simulink model "PEArray_func_sim"  (R2021a)
settings: Solver=VariableStepAuto  StartTime=0.0  StopTime=15  RelTol=1e-3
libraries: hdlBasic x164, xbsIndex_r4 x1
(part 1 of 2)
settings Model: Creator=lisix  LastModifiedBy=sl186
settings DebuggingCC: UnconnectedInputMsg=none  UnconnectedOutputMsg=none  UnconnectedLineMsg=none
settings RTWCC: DLArmComputeVersion=20.02.1

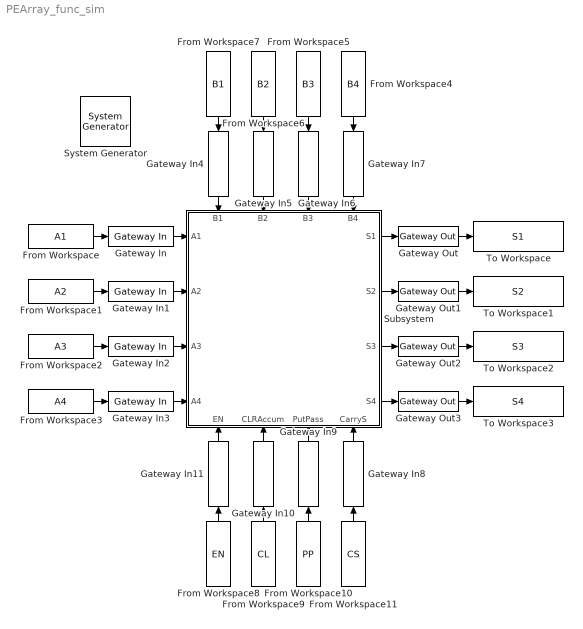
== system PEArray_func_sim ==
  " System Generator" : xbsIndex_r4/ System Generator  Tag=genX  xilinxfamily=zynq  part=xc7z020  speed=-1  package=clg484  synthesis_tool=Vivado  clock_wrapper=Clock Enables  directory=./netlist  proj_type=Vivado  Synth_file=Vivado Synthesis Defaults  Impl_file=Vivado Implementation Defaults  testbench=off  simulink_period=1  sysclk_period=10  dcm_input_clock_period=10  incr_netlist=off  trim_vbits=Everywhere in SubSystem  dbl_ovrd=According to Block Masks  core_generation=According to Block Masks  run_coregen=off  deprecated_control=off  eval_field=0  block_type=sysgen
  From Workspace : FromWorkspace  VariableName=A1  OutputAfterFinalValue=Setting to zero
  From Workspace1 : FromWorkspace  VariableName=A2  OutputAfterFinalValue=Setting to zero
  From Workspace10 : FromWorkspace  VariableName=PP  OutputAfterFinalValue=Setting to zero
  From Workspace11 : FromWorkspace  VariableName=CS  OutputAfterFinalValue=Setting to zero
  From Workspace2 : FromWorkspace  VariableName=A3  OutputAfterFinalValue=Setting to zero
  From Workspace3 : FromWorkspace  VariableName=A4  OutputAfterFinalValue=Setting to zero
  From Workspace4 : FromWorkspace  VariableName=B4  OutputAfterFinalValue=Setting to zero
  From Workspace5 : FromWorkspace  VariableName=B3  OutputAfterFinalValue=Setting to zero
  From Workspace6 : FromWorkspace  VariableName=B2  OutputAfterFinalValue=Setting to zero
  From Workspace7 : FromWorkspace  VariableName=B1  OutputAfterFinalValue=Setting to zero
  From Workspace8 : FromWorkspace  VariableName=EN  OutputAfterFinalValue=Setting to zero
  From Workspace9 : FromWorkspace  VariableName=CL  OutputAfterFinalValue=Setting to zero
  Gateway In{,1..7} (8 alike) : hdlBasic/Gateway In  gui_display_data_type=Fixed-point  arith_type=Signed (2's comp)  n_bits=16  bin_pt=10  preci_type=Single  exp_width=8  frac_width=24  rows=1  columns=1  quantization="Round  (unbiased: +/- Inf)"  overflow=Saturate  period=1  UseAsADC=off  ADCChannel='1'  interface=None  automatic_assignment=on  address_offset=hex2dec('00')  intf_name=''  intf_description=''  default_value=0  timing_constraint=None  locs_specified=off  LOCs={}  io_standard={}  inherit_from_input=off  hdl_port=on  XmcBlockStatus=1  maskContainerNames=group4  block_type=gatewayin  block_config=sysgen:gateway_in_config  block_width_w=590  block_height_w=620  block_width=640  block_height=850
  Gateway In{8..11} (4 alike) : hdlBasic/Gateway In  gui_display_data_type=Boolean  arith_type=Boolean  n_bits=16  bin_pt=10  preci_type=Single  exp_width=8  frac_width=24  rows=1  columns=1  quantization="Round  (unbiased: +/- Inf)"  overflow=Saturate  period=1  UseAsADC=off  ADCChannel='1'  interface=None  automatic_assignment=on  address_offset=hex2dec('00')  intf_name=''  intf_description=''  default_value=0  timing_constraint=None  locs_specified=off  LOCs={}  io_standard={}  inherit_from_input=off  hdl_port=on  XmcBlockStatus=1  maskContainerNames=group4  block_type=gatewayin  block_config=sysgen:gateway_in_config  block_width_w=590  block_height_w=620  block_width=640  block_height=850
  Gateway Out{,1..3} (4 alike) : hdlBasic/Gateway Out  inherit_from_input=off  hdl_port=on  rows=1  columns=1  UseAsDAC=off  DACChannel='1'  interface=None  automatic_assignment=on  address_offset=hex2dec('00')  intf_name=''  intf_description=''  timing_constraint=None  locs_specified=off  LOCs={}  io_standard={}  XmcBlockStatus=1  maskContainerNames=group4  block_type=gatewayout  block_config=sysgen:gateway_out_config  block_width_w=590  block_height_w=620  block_width=620  block_height=750
  Subsystem : Subsystem
      settings: PortSchema="{\"entries\":[{\"content\":{\"sides\":[{\"content\":{\"connectorIds\":[\"In1\",\"In2\",\"In3\",\"In4\"]},\"type\":\"ConnectorPlacement.EquallySpacedRectSide\",\"uuid\":\"ef644a02-469b-4d5d-af2f-26c489a3c425\"},{\"content\":{\"connectorIds\":[\"Out1\",\"Out2\",\"Out3\",\"Out4\"],\"side\":\"RIGHT\"},\"type\":\"ConnectorPlacement.EquallySpacedRectSide\",\"uuid\":\"314a2994-7795-41ba-894c-92e5f23e8912\"},{\"content\":{\"connectorIds\":[\"In5\",\"In6\",\"In7\",\"In8\"],\"side\":\"TOP\"},\"type\":\"ConnectorPlacement.EquallySpacedRectSide\",\"uuid\":\"0fc87e02-f682-470c-ba3d-89d91916b1fa\"},{\"content\":{\"connectorIds\":[\"In9\",\"In10\",\"In11\",\"In12\"],\"side\":\"BOTTOM\"},\"type\":\"ConnectorPlacement.EquallySpacedRectSide\",\"uuid\":\"d64b1621-eab0-4c50-9294-0c88aed07ecf\"}]},\"type\":\"ConnectorPlacement.EquallySpacedConnector\",\"uuid\":\"b7a51112-d4eb-4f46-8167-08a9d75329ad\"}],\"packageUris\":[\"http://schema.mathworks.com/mf0/Connector/R2020b\"],\"version\":\"1.0\"}"
  To Workspace : ToWorkspace  VariableName=S1  SaveFormat=Timeseries  SampleTime=-1
  To Workspace1 : ToWorkspace  VariableName=S2  SaveFormat=Timeseries  SampleTime=-1
  To Workspace2 : ToWorkspace  VariableName=S3  SaveFormat=Timeseries  SampleTime=-1
  To Workspace3 : ToWorkspace  VariableName=S4  SaveFormat=Timeseries  SampleTime=-1
  wires:
  Subsystem/1(S1) -> Gateway Out/1
  Subsystem/2(S2) -> Gateway Out1/1
  Subsystem/4(S4) -> Gateway Out3/1
  Subsystem/3(S3) -> Gateway Out2/1
  Gateway In/1 -> Subsystem/1(A1)
  Gateway In1/1 -> Subsystem/2(A2)
  Gateway In2/1 -> Subsystem/3(A3)
  Gateway In3/1 -> Subsystem/4(A4)
  Gateway In4/1 -> Subsystem/5(B1)
  Gateway In5/1 -> Subsystem/6(B2)
  Gateway In6/1 -> Subsystem/7(B3)
  Gateway In7/1 -> Subsystem/8(B4)
  From Workspace/1 -> Gateway In/1
  Gateway In11/1 -> Subsystem/9(EN)
  Gateway In10/1 -> Subsystem/10(CLRAccum)
  Gateway In9/1 -> Subsystem/11(PutPass)
  Gateway In8/1 -> Subsystem/12(CarryS)
  Gateway Out/1 -> To Workspace/1
  Gateway Out1/1 -> To Workspace1/1
  Gateway Out2/1 -> To Workspace2/1
  Gateway Out3/1 -> To Workspace3/1
  From Workspace1/1 -> Gateway In1/1
  From Workspace2/1 -> Gateway In2/1
  From Workspace3/1 -> Gateway In3/1
  From Workspace7/1 -> Gateway In4/1
  From Workspace6/1 -> Gateway In5/1
  From Workspace5/1 -> Gateway In6/1
  From Workspace4/1 -> Gateway In7/1
  From Workspace8/1 -> Gateway In11/1
  From Workspace9/1 -> Gateway In10/1
  From Workspace10/1 -> Gateway In9/1
  From Workspace11/1 -> Gateway In8/1

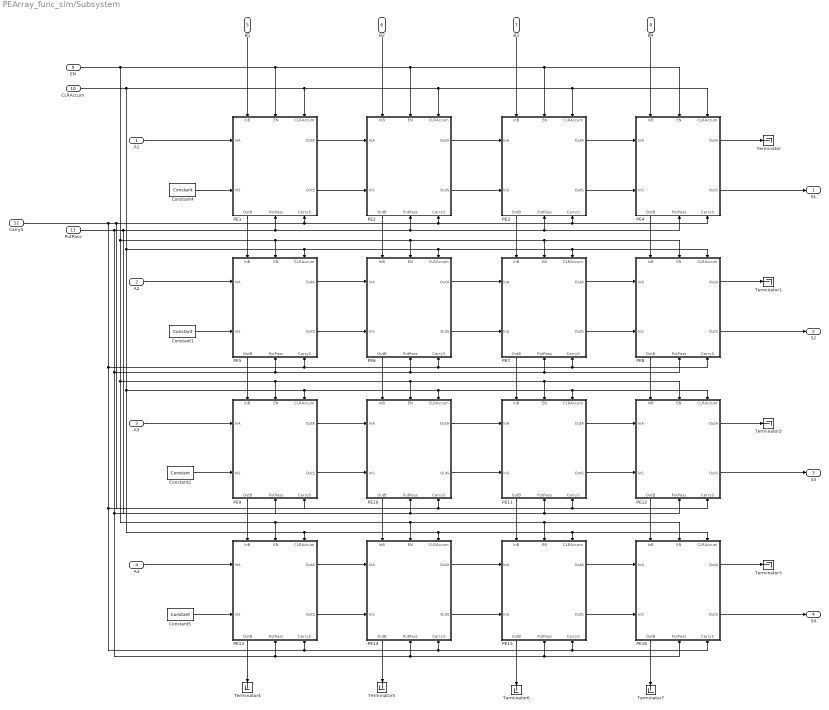
== system PEArray_func_sim/Subsystem ==
  A1 : Inport
  A2 : Inport  Port=2
  A3 : Inport  Port=3
  A4 : Inport  Port=4
  B1 : Inport  Port=5
  B2 : Inport  Port=6
  B3 : Inport  Port=7
  B4 : Inport  Port=8
  EN : Inport  Port=9
  CLRAccum : Inport  Port=10
  PutPass : Inport  Port=11
  CarryS : Inport  Port=12
  Constant{1..2,4..5} (4 alike) : hdlBasic/Constant  const=0  gui_display_data_type=Fixed-point  arith_type=Signed (2's comp)  n_bits=16  bin_pt=10  preci_type=Single  exp_width=8  frac_width=24  explicit_period=off  period=1  XmcBlockStatus=1  maskContainerNames=tabcontainer1  block_type=constant  block_config=sysgen:Constant_config
  PE1 : Subsystem
      settings: PortSchema="{\"entries\":[{\"content\":{\"sides\":[{\"content\":{\"connectorIds\":[\"In1\",\"In2\"]},\"type\":\"ConnectorPlacement.EquallySpacedRectSide\",\"uuid\":\"b0207bf0-c65c-4ff4-8705-318d6fed8092\"},{\"content\":{\"connectorIds\":[\"Out1\",\"Out2\"],\"side\":\"RIGHT\"},\"type\":\"ConnectorPlacement.EquallySpacedRectSide\",\"uuid\":\"a3adecdb-9d7d-41ad-9a9b-cd1de20cea82\"},{\"content\":{\"connectorIds\":[\"In3\",\"In4\",\"In5\"],\"side\":\"TOP\"},\"type\":\"ConnectorPlacement.EquallySpacedRectSide\",\"uuid\":\"b58b5fb8-8325-418d-b750-caf6dfdc9194\"},{\"content\":{\"connectorIds\":[\"Out3\",\"In6\",\"In7\"],\"side\":\"BOTTOM\"},\"type\":\"ConnectorPlacement.EquallySpacedRectSide\",\"uuid\":\"5c0ce549-850d-4243-a707-c43831315b10\"}]},\"type\":\"ConnectorPlacement.EquallySpacedConnector\",\"uuid\":\"239fabfc-6174-4768-8beb-49761318e2d6\"}],\"packageUris\":[\"http://schema.mathworks.com/mf0/Connector/R2020b\"],\"version\":\"1.0\"}"
  PE10 : Subsystem
      settings: PortSchema="{\"entries\":[{\"content\":{\"sides\":[{\"content\":{\"connectorIds\":[\"In1\",\"In2\"]},\"type\":\"ConnectorPlacement.EquallySpacedRectSide\",\"uuid\":\"b0207bf0-c65c-4ff4-8705-318d6fed8092\"},{\"content\":{\"connectorIds\":[\"Out1\",\"Out2\"],\"side\":\"RIGHT\"},\"type\":\"ConnectorPlacement.EquallySpacedRectSide\",\"uuid\":\"a3adecdb-9d7d-41ad-9a9b-cd1de20cea82\"},{\"content\":{\"connectorIds\":[\"In3\",\"In4\",\"In5\"],\"side\":\"TOP\"},\"type\":\"ConnectorPlacement.EquallySpacedRectSide\",\"uuid\":\"b58b5fb8-8325-418d-b750-caf6dfdc9194\"},{\"content\":{\"connectorIds\":[\"Out3\",\"In6\",\"In7\"],\"side\":\"BOTTOM\"},\"type\":\"ConnectorPlacement.EquallySpacedRectSide\",\"uuid\":\"5c0ce549-850d-4243-a707-c43831315b10\"}]},\"type\":\"ConnectorPlacement.EquallySpacedConnector\",\"uuid\":\"239fabfc-6174-4768-8beb-49761318e2d6\"}],\"packageUris\":[\"http://schema.mathworks.com/mf0/Connector/R2020b\"],\"version\":\"1.0\"}"
  PE11 : Subsystem
      settings: PortSchema="{\"entries\":[{\"content\":{\"sides\":[{\"content\":{\"connectorIds\":[\"In1\",\"In2\"]},\"type\":\"ConnectorPlacement.EquallySpacedRectSide\",\"uuid\":\"b0207bf0-c65c-4ff4-8705-318d6fed8092\"},{\"content\":{\"connectorIds\":[\"Out1\",\"Out2\"],\"side\":\"RIGHT\"},\"type\":\"ConnectorPlacement.EquallySpacedRectSide\",\"uuid\":\"a3adecdb-9d7d-41ad-9a9b-cd1de20cea82\"},{\"content\":{\"connectorIds\":[\"In3\",\"In4\",\"In5\"],\"side\":\"TOP\"},\"type\":\"ConnectorPlacement.EquallySpacedRectSide\",\"uuid\":\"b58b5fb8-8325-418d-b750-caf6dfdc9194\"},{\"content\":{\"connectorIds\":[\"Out3\",\"In6\",\"In7\"],\"side\":\"BOTTOM\"},\"type\":\"ConnectorPlacement.EquallySpacedRectSide\",\"uuid\":\"5c0ce549-850d-4243-a707-c43831315b10\"}]},\"type\":\"ConnectorPlacement.EquallySpacedConnector\",\"uuid\":\"239fabfc-6174-4768-8beb-49761318e2d6\"}],\"packageUris\":[\"http://schema.mathworks.com/mf0/Connector/R2020b\"],\"version\":\"1.0\"}"
  PE12 : Subsystem
      settings: PortSchema="{\"entries\":[{\"content\":{\"sides\":[{\"content\":{\"connectorIds\":[\"In1\",\"In2\"]},\"type\":\"ConnectorPlacement.EquallySpacedRectSide\",\"uuid\":\"b0207bf0-c65c-4ff4-8705-318d6fed8092\"},{\"content\":{\"connectorIds\":[\"Out1\",\"Out2\"],\"side\":\"RIGHT\"},\"type\":\"ConnectorPlacement.EquallySpacedRectSide\",\"uuid\":\"a3adecdb-9d7d-41ad-9a9b-cd1de20cea82\"},{\"content\":{\"connectorIds\":[\"In3\",\"In4\",\"In5\"],\"side\":\"TOP\"},\"type\":\"ConnectorPlacement.EquallySpacedRectSide\",\"uuid\":\"b58b5fb8-8325-418d-b750-caf6dfdc9194\"},{\"content\":{\"connectorIds\":[\"Out3\",\"In6\",\"In7\"],\"side\":\"BOTTOM\"},\"type\":\"ConnectorPlacement.EquallySpacedRectSide\",\"uuid\":\"5c0ce549-850d-4243-a707-c43831315b10\"}]},\"type\":\"ConnectorPlacement.EquallySpacedConnector\",\"uuid\":\"239fabfc-6174-4768-8beb-49761318e2d6\"}],\"packageUris\":[\"http://schema.mathworks.com/mf0/Connector/R2020b\"],\"version\":\"1.0\"}"
  PE13 : Subsystem
      settings: PortSchema="{\"entries\":[{\"content\":{\"sides\":[{\"content\":{\"connectorIds\":[\"In1\",\"In2\"]},\"type\":\"ConnectorPlacement.EquallySpacedRectSide\",\"uuid\":\"b0207bf0-c65c-4ff4-8705-318d6fed8092\"},{\"content\":{\"connectorIds\":[\"Out1\",\"Out2\"],\"side\":\"RIGHT\"},\"type\":\"ConnectorPlacement.EquallySpacedRectSide\",\"uuid\":\"a3adecdb-9d7d-41ad-9a9b-cd1de20cea82\"},{\"content\":{\"connectorIds\":[\"In3\",\"In4\",\"In5\"],\"side\":\"TOP\"},\"type\":\"ConnectorPlacement.EquallySpacedRectSide\",\"uuid\":\"b58b5fb8-8325-418d-b750-caf6dfdc9194\"},{\"content\":{\"connectorIds\":[\"Out3\",\"In6\",\"In7\"],\"side\":\"BOTTOM\"},\"type\":\"ConnectorPlacement.EquallySpacedRectSide\",\"uuid\":\"5c0ce549-850d-4243-a707-c43831315b10\"}]},\"type\":\"ConnectorPlacement.EquallySpacedConnector\",\"uuid\":\"239fabfc-6174-4768-8beb-49761318e2d6\"}],\"packageUris\":[\"http://schema.mathworks.com/mf0/Connector/R2020b\"],\"version\":\"1.0\"}"
  PE14 : Subsystem
      settings: PortSchema="{\"entries\":[{\"content\":{\"sides\":[{\"content\":{\"connectorIds\":[\"In1\",\"In2\"]},\"type\":\"ConnectorPlacement.EquallySpacedRectSide\",\"uuid\":\"b0207bf0-c65c-4ff4-8705-318d6fed8092\"},{\"content\":{\"connectorIds\":[\"Out1\",\"Out2\"],\"side\":\"RIGHT\"},\"type\":\"ConnectorPlacement.EquallySpacedRectSide\",\"uuid\":\"a3adecdb-9d7d-41ad-9a9b-cd1de20cea82\"},{\"content\":{\"connectorIds\":[\"In3\",\"In4\",\"In5\"],\"side\":\"TOP\"},\"type\":\"ConnectorPlacement.EquallySpacedRectSide\",\"uuid\":\"b58b5fb8-8325-418d-b750-caf6dfdc9194\"},{\"content\":{\"connectorIds\":[\"Out3\",\"In6\",\"In7\"],\"side\":\"BOTTOM\"},\"type\":\"ConnectorPlacement.EquallySpacedRectSide\",\"uuid\":\"5c0ce549-850d-4243-a707-c43831315b10\"}]},\"type\":\"ConnectorPlacement.EquallySpacedConnector\",\"uuid\":\"239fabfc-6174-4768-8beb-49761318e2d6\"}],\"packageUris\":[\"http://schema.mathworks.com/mf0/Connector/R2020b\"],\"version\":\"1.0\"}"
  PE15 : Subsystem
      settings: PortSchema="{\"entries\":[{\"content\":{\"sides\":[{\"content\":{\"connectorIds\":[\"In1\",\"In2\"]},\"type\":\"ConnectorPlacement.EquallySpacedRectSide\",\"uuid\":\"b0207bf0-c65c-4ff4-8705-318d6fed8092\"},{\"content\":{\"connectorIds\":[\"Out1\",\"Out2\"],\"side\":\"RIGHT\"},\"type\":\"ConnectorPlacement.EquallySpacedRectSide\",\"uuid\":\"a3adecdb-9d7d-41ad-9a9b-cd1de20cea82\"},{\"content\":{\"connectorIds\":[\"In3\",\"In4\",\"In5\"],\"side\":\"TOP\"},\"type\":\"ConnectorPlacement.EquallySpacedRectSide\",\"uuid\":\"b58b5fb8-8325-418d-b750-caf6dfdc9194\"},{\"content\":{\"connectorIds\":[\"Out3\",\"In6\",\"In7\"],\"side\":\"BOTTOM\"},\"type\":\"ConnectorPlacement.EquallySpacedRectSide\",\"uuid\":\"5c0ce549-850d-4243-a707-c43831315b10\"}]},\"type\":\"ConnectorPlacement.EquallySpacedConnector\",\"uuid\":\"239fabfc-6174-4768-8beb-49761318e2d6\"}],\"packageUris\":[\"http://schema.mathworks.com/mf0/Connector/R2020b\"],\"version\":\"1.0\"}"
  PE16 : Subsystem
      settings: PortSchema="{\"entries\":[{\"content\":{\"sides\":[{\"content\":{\"connectorIds\":[\"In1\",\"In2\"]},\"type\":\"ConnectorPlacement.EquallySpacedRectSide\",\"uuid\":\"b0207bf0-c65c-4ff4-8705-318d6fed8092\"},{\"content\":{\"connectorIds\":[\"Out1\",\"Out2\"],\"side\":\"RIGHT\"},\"type\":\"ConnectorPlacement.EquallySpacedRectSide\",\"uuid\":\"a3adecdb-9d7d-41ad-9a9b-cd1de20cea82\"},{\"content\":{\"connectorIds\":[\"In3\",\"In4\",\"In5\"],\"side\":\"TOP\"},\"type\":\"ConnectorPlacement.EquallySpacedRectSide\",\"uuid\":\"b58b5fb8-8325-418d-b750-caf6dfdc9194\"},{\"content\":{\"connectorIds\":[\"Out3\",\"In6\",\"In7\"],\"side\":\"BOTTOM\"},\"type\":\"ConnectorPlacement.EquallySpacedRectSide\",\"uuid\":\"5c0ce549-850d-4243-a707-c43831315b10\"}]},\"type\":\"ConnectorPlacement.EquallySpacedConnector\",\"uuid\":\"239fabfc-6174-4768-8beb-49761318e2d6\"}],\"packageUris\":[\"http://schema.mathworks.com/mf0/Connector/R2020b\"],\"version\":\"1.0\"}"
  PE2 : Subsystem
      settings: PortSchema="{\"entries\":[{\"content\":{\"sides\":[{\"content\":{\"connectorIds\":[\"In1\",\"In2\"]},\"type\":\"ConnectorPlacement.EquallySpacedRectSide\",\"uuid\":\"b0207bf0-c65c-4ff4-8705-318d6fed8092\"},{\"content\":{\"connectorIds\":[\"Out1\",\"Out2\"],\"side\":\"RIGHT\"},\"type\":\"ConnectorPlacement.EquallySpacedRectSide\",\"uuid\":\"a3adecdb-9d7d-41ad-9a9b-cd1de20cea82\"},{\"content\":{\"connectorIds\":[\"In3\",\"In4\",\"In5\"],\"side\":\"TOP\"},\"type\":\"ConnectorPlacement.EquallySpacedRectSide\",\"uuid\":\"b58b5fb8-8325-418d-b750-caf6dfdc9194\"},{\"content\":{\"connectorIds\":[\"Out3\",\"In6\",\"In7\"],\"side\":\"BOTTOM\"},\"type\":\"ConnectorPlacement.EquallySpacedRectSide\",\"uuid\":\"5c0ce549-850d-4243-a707-c43831315b10\"}]},\"type\":\"ConnectorPlacement.EquallySpacedConnector\",\"uuid\":\"239fabfc-6174-4768-8beb-49761318e2d6\"}],\"packageUris\":[\"http://schema.mathworks.com/mf0/Connector/R2020b\"],\"version\":\"1.0\"}"
  PE3 : Subsystem
      settings: PortSchema="{\"entries\":[{\"content\":{\"sides\":[{\"content\":{\"connectorIds\":[\"In1\",\"In2\"]},\"type\":\"ConnectorPlacement.EquallySpacedRectSide\",\"uuid\":\"b0207bf0-c65c-4ff4-8705-318d6fed8092\"},{\"content\":{\"connectorIds\":[\"Out1\",\"Out2\"],\"side\":\"RIGHT\"},\"type\":\"ConnectorPlacement.EquallySpacedRectSide\",\"uuid\":\"a3adecdb-9d7d-41ad-9a9b-cd1de20cea82\"},{\"content\":{\"connectorIds\":[\"In3\",\"In4\",\"In5\"],\"side\":\"TOP\"},\"type\":\"ConnectorPlacement.EquallySpacedRectSide\",\"uuid\":\"b58b5fb8-8325-418d-b750-caf6dfdc9194\"},{\"content\":{\"connectorIds\":[\"Out3\",\"In6\",\"In7\"],\"side\":\"BOTTOM\"},\"type\":\"ConnectorPlacement.EquallySpacedRectSide\",\"uuid\":\"5c0ce549-850d-4243-a707-c43831315b10\"}]},\"type\":\"ConnectorPlacement.EquallySpacedConnector\",\"uuid\":\"239fabfc-6174-4768-8beb-49761318e2d6\"}],\"packageUris\":[\"http://schema.mathworks.com/mf0/Connector/R2020b\"],\"version\":\"1.0\"}"
  PE4 : Subsystem
      settings: PortSchema="{\"entries\":[{\"content\":{\"sides\":[{\"content\":{\"connectorIds\":[\"In1\",\"In2\"]},\"type\":\"ConnectorPlacement.EquallySpacedRectSide\",\"uuid\":\"b0207bf0-c65c-4ff4-8705-318d6fed8092\"},{\"content\":{\"connectorIds\":[\"Out1\",\"Out2\"],\"side\":\"RIGHT\"},\"type\":\"ConnectorPlacement.EquallySpacedRectSide\",\"uuid\":\"a3adecdb-9d7d-41ad-9a9b-cd1de20cea82\"},{\"content\":{\"connectorIds\":[\"In3\",\"In4\",\"In5\"],\"side\":\"TOP\"},\"type\":\"ConnectorPlacement.EquallySpacedRectSide\",\"uuid\":\"b58b5fb8-8325-418d-b750-caf6dfdc9194\"},{\"content\":{\"connectorIds\":[\"Out3\",\"In6\",\"In7\"],\"side\":\"BOTTOM\"},\"type\":\"ConnectorPlacement.EquallySpacedRectSide\",\"uuid\":\"5c0ce549-850d-4243-a707-c43831315b10\"}]},\"type\":\"ConnectorPlacement.EquallySpacedConnector\",\"uuid\":\"239fabfc-6174-4768-8beb-49761318e2d6\"}],\"packageUris\":[\"http://schema.mathworks.com/mf0/Connector/R2020b\"],\"version\":\"1.0\"}"
  PE5 : Subsystem
      settings: PortSchema="{\"entries\":[{\"content\":{\"sides\":[{\"content\":{\"connectorIds\":[\"In1\",\"In2\"]},\"type\":\"ConnectorPlacement.EquallySpacedRectSide\",\"uuid\":\"b0207bf0-c65c-4ff4-8705-318d6fed8092\"},{\"content\":{\"connectorIds\":[\"Out1\",\"Out2\"],\"side\":\"RIGHT\"},\"type\":\"ConnectorPlacement.EquallySpacedRectSide\",\"uuid\":\"a3adecdb-9d7d-41ad-9a9b-cd1de20cea82\"},{\"content\":{\"connectorIds\":[\"In3\",\"In4\",\"In5\"],\"side\":\"TOP\"},\"type\":\"ConnectorPlacement.EquallySpacedRectSide\",\"uuid\":\"b58b5fb8-8325-418d-b750-caf6dfdc9194\"},{\"content\":{\"connectorIds\":[\"Out3\",\"In6\",\"In7\"],\"side\":\"BOTTOM\"},\"type\":\"ConnectorPlacement.EquallySpacedRectSide\",\"uuid\":\"5c0ce549-850d-4243-a707-c43831315b10\"}]},\"type\":\"ConnectorPlacement.EquallySpacedConnector\",\"uuid\":\"239fabfc-6174-4768-8beb-49761318e2d6\"}],\"packageUris\":[\"http://schema.mathworks.com/mf0/Connector/R2020b\"],\"version\":\"1.0\"}"
  PE6 : Subsystem
      settings: PortSchema="{\"entries\":[{\"content\":{\"sides\":[{\"content\":{\"connectorIds\":[\"In1\",\"In2\"]},\"type\":\"ConnectorPlacement.EquallySpacedRectSide\",\"uuid\":\"b0207bf0-c65c-4ff4-8705-318d6fed8092\"},{\"content\":{\"connectorIds\":[\"Out1\",\"Out2\"],\"side\":\"RIGHT\"},\"type\":\"ConnectorPlacement.EquallySpacedRectSide\",\"uuid\":\"a3adecdb-9d7d-41ad-9a9b-cd1de20cea82\"},{\"content\":{\"connectorIds\":[\"In3\",\"In4\",\"In5\"],\"side\":\"TOP\"},\"type\":\"ConnectorPlacement.EquallySpacedRectSide\",\"uuid\":\"b58b5fb8-8325-418d-b750-caf6dfdc9194\"},{\"content\":{\"connectorIds\":[\"Out3\",\"In6\",\"In7\"],\"side\":\"BOTTOM\"},\"type\":\"ConnectorPlacement.EquallySpacedRectSide\",\"uuid\":\"5c0ce549-850d-4243-a707-c43831315b10\"}]},\"type\":\"ConnectorPlacement.EquallySpacedConnector\",\"uuid\":\"239fabfc-6174-4768-8beb-49761318e2d6\"}],\"packageUris\":[\"http://schema.mathworks.com/mf0/Connector/R2020b\"],\"version\":\"1.0\"}"
  PE7 : Subsystem
      settings: PortSchema="{\"entries\":[{\"content\":{\"sides\":[{\"content\":{\"connectorIds\":[\"In1\",\"In2\"]},\"type\":\"ConnectorPlacement.EquallySpacedRectSide\",\"uuid\":\"b0207bf0-c65c-4ff4-8705-318d6fed8092\"},{\"content\":{\"connectorIds\":[\"Out1\",\"Out2\"],\"side\":\"RIGHT\"},\"type\":\"ConnectorPlacement.EquallySpacedRectSide\",\"uuid\":\"a3adecdb-9d7d-41ad-9a9b-cd1de20cea82\"},{\"content\":{\"connectorIds\":[\"In3\",\"In4\",\"In5\"],\"side\":\"TOP\"},\"type\":\"ConnectorPlacement.EquallySpacedRectSide\",\"uuid\":\"b58b5fb8-8325-418d-b750-caf6dfdc9194\"},{\"content\":{\"connectorIds\":[\"Out3\",\"In6\",\"In7\"],\"side\":\"BOTTOM\"},\"type\":\"ConnectorPlacement.EquallySpacedRectSide\",\"uuid\":\"5c0ce549-850d-4243-a707-c43831315b10\"}]},\"type\":\"ConnectorPlacement.EquallySpacedConnector\",\"uuid\":\"239fabfc-6174-4768-8beb-49761318e2d6\"}],\"packageUris\":[\"http://schema.mathworks.com/mf0/Connector/R2020b\"],\"version\":\"1.0\"}"
  PE8 : Subsystem
      settings: PortSchema="{\"entries\":[{\"content\":{\"sides\":[{\"content\":{\"connectorIds\":[\"In1\",\"In2\"]},\"type\":\"ConnectorPlacement.EquallySpacedRectSide\",\"uuid\":\"b0207bf0-c65c-4ff4-8705-318d6fed8092\"},{\"content\":{\"connectorIds\":[\"Out1\",\"Out2\"],\"side\":\"RIGHT\"},\"type\":\"ConnectorPlacement.EquallySpacedRectSide\",\"uuid\":\"a3adecdb-9d7d-41ad-9a9b-cd1de20cea82\"},{\"content\":{\"connectorIds\":[\"In3\",\"In4\",\"In5\"],\"side\":\"TOP\"},\"type\":\"ConnectorPlacement.EquallySpacedRectSide\",\"uuid\":\"b58b5fb8-8325-418d-b750-caf6dfdc9194\"},{\"content\":{\"connectorIds\":[\"Out3\",\"In6\",\"In7\"],\"side\":\"BOTTOM\"},\"type\":\"ConnectorPlacement.EquallySpacedRectSide\",\"uuid\":\"5c0ce549-850d-4243-a707-c43831315b10\"}]},\"type\":\"ConnectorPlacement.EquallySpacedConnector\",\"uuid\":\"239fabfc-6174-4768-8beb-49761318e2d6\"}],\"packageUris\":[\"http://schema.mathworks.com/mf0/Connector/R2020b\"],\"version\":\"1.0\"}"
  PE9 : Subsystem
      settings: PortSchema="{\"entries\":[{\"content\":{\"sides\":[{\"content\":{\"connectorIds\":[\"In1\",\"In2\"]},\"type\":\"ConnectorPlacement.EquallySpacedRectSide\",\"uuid\":\"b0207bf0-c65c-4ff4-8705-318d6fed8092\"},{\"content\":{\"connectorIds\":[\"Out1\",\"Out2\"],\"side\":\"RIGHT\"},\"type\":\"ConnectorPlacement.EquallySpacedRectSide\",\"uuid\":\"a3adecdb-9d7d-41ad-9a9b-cd1de20cea82\"},{\"content\":{\"connectorIds\":[\"In3\",\"In4\",\"In5\"],\"side\":\"TOP\"},\"type\":\"ConnectorPlacement.EquallySpacedRectSide\",\"uuid\":\"b58b5fb8-8325-418d-b750-caf6dfdc9194\"},{\"content\":{\"connectorIds\":[\"Out3\",\"In6\",\"In7\"],\"side\":\"BOTTOM\"},\"type\":\"ConnectorPlacement.EquallySpacedRectSide\",\"uuid\":\"5c0ce549-850d-4243-a707-c43831315b10\"}]},\"type\":\"ConnectorPlacement.EquallySpacedConnector\",\"uuid\":\"239fabfc-6174-4768-8beb-49761318e2d6\"}],\"packageUris\":[\"http://schema.mathworks.com/mf0/Connector/R2020b\"],\"version\":\"1.0\"}"
  Terminator{,1..7} (8 alike) : Terminator
  S1 : Outport
  S2 : Outport  Port=2
  S3 : Outport  Port=3
  S4 : Outport  Port=4
  wires:
  PE16/1(OutA) -> Terminator3/1
  PE3/3(OutB) -> PE7/3(InB)
  PE13/2(OutS) -> PE14/2(InS)
  PE5/1(OutA) -> PE6/1(InA)
  CLRAccum/1 -> PE8/5(CLRAccum), PE7/5(CLRAccum), PE6/5(CLRAccum), PE5/5(CLRAccum), PE12/5(CLRAccum), PE11/5(CLRAccum), PE10/5(CLRAccum), PE9/5(CLRAccum), PE16/5(CLRAccum), PE15/5(CLRAccum), PE14/5(CLRAccum), PE13/5(CLRAccum), PE4/5(CLRAccum), PE3/5(CLRAccum), PE2/5(CLRAccum), PE1/5(CLRAccum)
  EN/1 -> PE4/4(EN), PE3/4(EN), PE2/4(EN), PE1/4(EN), PE8/4(EN), PE7/4(EN), PE6/4(EN), PE5/4(EN), PE12/4(EN), PE11/4(EN), PE10/4(EN), PE9/4(EN), PE16/4(EN), PE15/4(EN), PE14/4(EN), PE13/4(EN)
  PE9/2(OutS) -> PE10/2(InS)
  PE9/1(OutA) -> PE10/1(InA)
  PE8/1(OutA) -> Terminator1/1
  PE11/3(OutB) -> PE15/3(InB)
  Constant5/1 -> PE13/2(InS)
  PE5/2(OutS) -> PE6/2(InS)
  B3/1 -> PE3/3(InB)
  Constant4/1 -> PE1/2(InS)
  PE7/3(OutB) -> PE11/3(InB)
  CarryS/1 -> PE4/7(CarryS), PE3/7(CarryS), PE2/7(CarryS), PE1/7(CarryS), PE12/7(CarryS), PE11/7(CarryS), PE10/7(CarryS), PE9/7(CarryS), PE16/7(CarryS), PE15/7(CarryS), PE14/7(CarryS), PE13/7(CarryS), PE8/7(CarryS), PE7/7(CarryS), PE6/7(CarryS), PE5/7(CarryS)
  PE6/3(OutB) -> PE10/3(InB)
  PutPass/1 -> PE11/6(PutPass), PE12/6(PutPass), PE10/6(PutPass), PE4/6(PutPass), PE3/6(PutPass), PE2/6(PutPass), PE1/6(PutPass), PE8/6(PutPass), PE7/6(PutPass), PE6/6(PutPass), PE5/6(PutPass), PE16/6(PutPass), PE15/6(PutPass), PE14/6(PutPass), PE13/6(PutPass), PE9/6(PutPass)
  PE2/1(OutA) -> PE3/1(InA)
  PE12/1(OutA) -> Terminator2/1
  A1/1 -> PE1/1(InA)
  PE11/1(OutA) -> PE12/1(InA)
  PE10/1(OutA) -> PE11/1(InA)
  PE1/2(OutS) -> PE2/2(InS)
  PE11/2(OutS) -> PE12/2(InS)
  PE10/2(OutS) -> PE11/2(InS)
  B4/1 -> PE4/3(InB)
  PE14/2(OutS) -> PE15/2(InS)
  Constant2/1 -> PE9/2(InS)
  PE10/3(OutB) -> PE14/3(InB)
  PE15/2(OutS) -> PE16/2(InS)
  PE14/1(OutA) -> PE15/1(InA)
  PE13/1(OutA) -> PE14/1(InA)
  PE15/1(OutA) -> PE16/1(InA)
  PE6/2(OutS) -> PE7/2(InS)
  PE12/3(OutB) -> PE16/3(InB)
  PE2/3(OutB) -> PE6/3(InB)
  PE7/1(OutA) -> PE8/1(InA)
  PE7/2(OutS) -> PE8/2(InS)
  PE9/3(OutB) -> PE13/3(InB)
  PE16/2(OutS) -> S4/1
  PE8/2(OutS) -> S2/1
  PE1/3(OutB) -> PE5/3(InB)
  PE4/1(OutA) -> Terminator/1
  PE4/2(OutS) -> S1/1
  B2/1 -> PE2/3(InB)
  Constant1/1 -> PE5/2(InS)
  PE3/2(OutS) -> PE4/2(InS)
  A3/1 -> PE9/1(InA)
  PE4/3(OutB) -> PE8/3(InB)
  B1/1 -> PE1/3(InB)
  A4/1 -> PE13/1(InA)
  A2/1 -> PE5/1(InA)
  PE6/1(OutA) -> PE7/1(InA)
  PE2/2(OutS) -> PE3/2(InS)
  PE3/1(OutA) -> PE4/1(InA)
  PE5/3(OutB) -> PE9/3(InB)
  PE1/1(OutA) -> PE2/1(InA)
  PE12/2(OutS) -> S3/1
  PE8/3(OutB) -> PE12/3(InB)
  PE13/3(OutB) -> Terminator4/1
  PE14/3(OutB) -> Terminator5/1
  PE15/3(OutB) -> Terminator6/1
  PE16/3(OutB) -> Terminator7/1

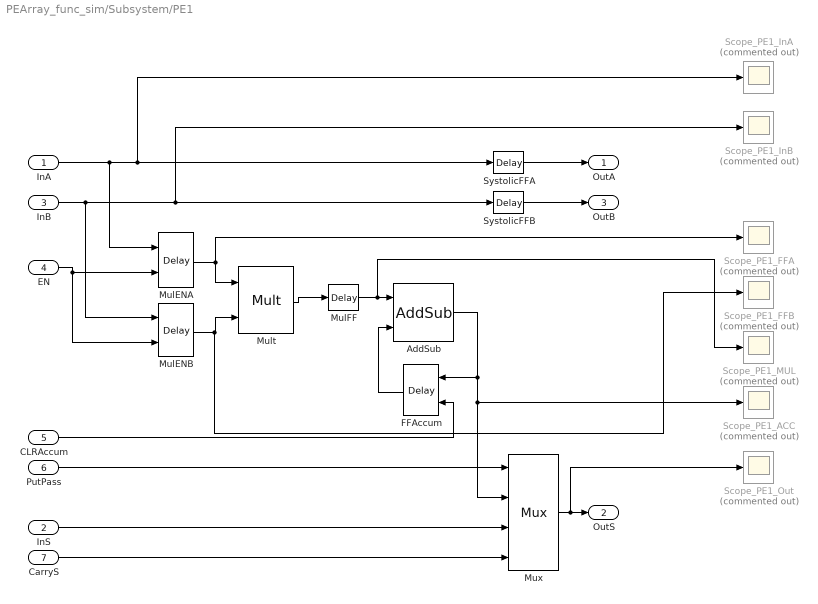
== system PEArray_func_sim/Subsystem/PE1 ==
  InA : Inport
  InS : Inport  Port=2
  InB : Inport  Port=3
  EN : Inport  Port=4
  CLRAccum : Inport  Port=5
  PutPass : Inport  Port=6
  CarryS : Inport  Port=7
  AddSub : hdlBasic/AddSub  mode=Addition  use_carryin=off  use_carryout=off  en=off  latency=0  precision=User Defined  arith_type="Signed  (2's comp)"  n_bits=16  bin_pt=10  quantization=Truncate  overflow=Wrap  use_behavioral_HDL=off  hw_selection=DSP48  pipelined=off  XmcBlockStatus=1  maskContainerNames=tabcontainer1  block_type=addsub  block_config=sysgen:Addsub_config
  FFAccum : hdlBasic/Delay  rst=on  en=off  latency=1  reg_retiming=off  XmcBlockStatus=1  maskContainerNames=group1  block_type=delay  block_config=sysgen:Delay_config
  MulENA : hdlBasic/Delay  rst=on  en=off  latency=1  reg_retiming=off  XmcBlockStatus=1  maskContainerNames=group1  block_type=delay  block_config=sysgen:Delay_config
  MulENB : hdlBasic/Delay  rst=on  en=off  latency=1  reg_retiming=off  XmcBlockStatus=1  maskContainerNames=group1  block_type=delay  block_config=sysgen:Delay_config
  MulFF : hdlBasic/Delay  rst=off  en=off  latency=1  reg_retiming=off  XmcBlockStatus=1  maskContainerNames=group1  block_type=delay  block_config=sysgen:Delay_config
  Mult : hdlBasic/Mult  precision=User Defined  arith_type="Signed  (2's comp)"  n_bits=16  bin_pt=10  quantization=Truncate  overflow=Wrap  en=off  latency=0  use_behavioral_HDL=off  opt=Speed  use_embedded=on  optimum_pipeline=off  pipeline=on  use_rpm=on  placement_style=Triangular  XmcBlockStatus=1  maskContainerNames=group1  block_type=mult  block_config=sysgen:Mult_config
  Mux : hdlBasic/Mux  inputs=2  en=on  latency=1  precision=Full  arith_type=Unsigned  n_bits=16  bin_pt=14  quantization=Truncate  overflow=Wrap  XmcBlockStatus=1  maskContainerNames=tabcontainer1  block_type=mux  block_config=sysgen:Mux_config
  Scope_PE1_ACC : Scope  Commented=on
  Scope_PE1_FFA : Scope  Commented=on
  Scope_PE1_FFB : Scope  Commented=on
  Scope_PE1_InA : Scope  Commented=on
  Scope_PE1_InB : Scope  Commented=on
  Scope_PE1_MUL : Scope  Commented=on
  Scope_PE1_Out : Scope  Commented=on
  SystolicFFA : hdlBasic/Delay  rst=off  en=off  latency=1  reg_retiming=off  XmcBlockStatus=1  maskContainerNames=group1  block_type=delay  block_config=sysgen:Delay_config
  SystolicFFB : hdlBasic/Delay  rst=off  en=off  latency=1  reg_retiming=off  XmcBlockStatus=1  maskContainerNames=group1  block_type=delay  block_config=sysgen:Delay_config
  OutA : Outport
  OutS : Outport  Port=2
  OutB : Outport  Port=3
  wires:
  Mult/1 -> MulFF/1
  MulFF/1 -> Scope_PE1_MUL/1, AddSub/1
  AddSub/1 -> Scope_PE1_ACC/1, Mux/2, FFAccum/1
  InB/1 -> MulENB/1, Scope_PE1_InB/1, SystolicFFB/1
  InA/1 -> MulENA/1, Scope_PE1_InA/1, SystolicFFA/1
  SystolicFFB/1 -> OutB/1
  SystolicFFA/1 -> OutA/1
  MulENA/1 -> Mult/1, Scope_PE1_FFA/1
  MulENB/1 -> Scope_PE1_FFB/1, Mult/2
  EN/1 -> MulENB/2, MulENA/2
  FFAccum/1 -> AddSub/2
  CLRAccum/1 -> FFAccum/2
  PutPass/1 -> Mux/1
  InS/1 -> Mux/3
  Mux/1 -> Scope_PE1_Out/1, OutS/1
  CarryS/1 -> Mux/4

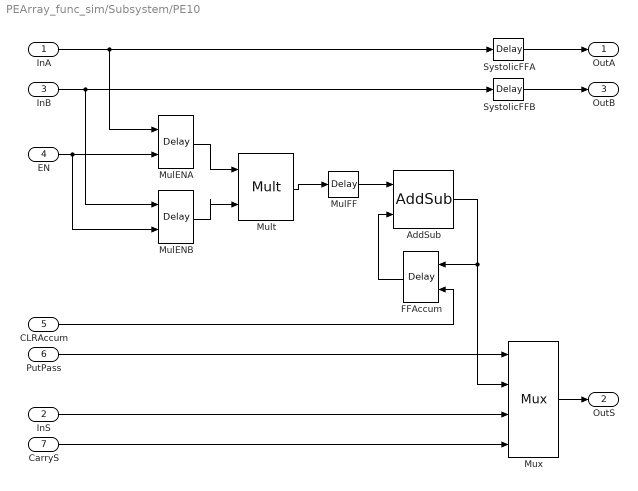
== system PEArray_func_sim/Subsystem/PE10 ==
  InA : Inport
  InS : Inport  Port=2
  InB : Inport  Port=3
  EN : Inport  Port=4
  CLRAccum : Inport  Port=5
  PutPass : Inport  Port=6
  CarryS : Inport  Port=7
  AddSub : hdlBasic/AddSub  mode=Addition  use_carryin=off  use_carryout=off  en=off  latency=0  precision=User Defined  arith_type="Signed  (2's comp)"  n_bits=16  bin_pt=10  quantization=Truncate  overflow=Wrap  use_behavioral_HDL=off  hw_selection=DSP48  pipelined=off  XmcBlockStatus=1  maskContainerNames=tabcontainer1  block_type=addsub  block_config=sysgen:Addsub_config
  FFAccum : hdlBasic/Delay  rst=on  en=off  latency=1  reg_retiming=off  XmcBlockStatus=1  maskContainerNames=group1  block_type=delay  block_config=sysgen:Delay_config
  MulENA : hdlBasic/Delay  rst=on  en=off  latency=1  reg_retiming=off  XmcBlockStatus=1  maskContainerNames=group1  block_type=delay  block_config=sysgen:Delay_config
  MulENB : hdlBasic/Delay  rst=on  en=off  latency=1  reg_retiming=off  XmcBlockStatus=1  maskContainerNames=group1  block_type=delay  block_config=sysgen:Delay_config
  MulFF : hdlBasic/Delay  rst=off  en=off  latency=1  reg_retiming=off  XmcBlockStatus=1  maskContainerNames=group1  block_type=delay  block_config=sysgen:Delay_config
  Mult : hdlBasic/Mult  precision=User Defined  arith_type="Signed  (2's comp)"  n_bits=16  bin_pt=10  quantization=Truncate  overflow=Wrap  en=off  latency=0  use_behavioral_HDL=off  opt=Speed  use_embedded=on  optimum_pipeline=off  pipeline=on  use_rpm=on  placement_style=Triangular  XmcBlockStatus=1  maskContainerNames=group1  block_type=mult  block_config=sysgen:Mult_config
  Mux : hdlBasic/Mux  inputs=2  en=on  latency=1  precision=Full  arith_type=Unsigned  n_bits=16  bin_pt=14  quantization=Truncate  overflow=Wrap  XmcBlockStatus=1  maskContainerNames=tabcontainer1  block_type=mux  block_config=sysgen:Mux_config
  SystolicFFA : hdlBasic/Delay  rst=off  en=off  latency=1  reg_retiming=off  XmcBlockStatus=1  maskContainerNames=group1  block_type=delay  block_config=sysgen:Delay_config
  SystolicFFB : hdlBasic/Delay  rst=off  en=off  latency=1  reg_retiming=off  XmcBlockStatus=1  maskContainerNames=group1  block_type=delay  block_config=sysgen:Delay_config
  OutA : Outport
  OutS : Outport  Port=2
  OutB : Outport  Port=3
  wires:
  Mult/1 -> MulFF/1
  MulFF/1 -> AddSub/1
  AddSub/1 -> Mux/2, FFAccum/1
  InB/1 -> MulENB/1, SystolicFFB/1
  InA/1 -> MulENA/1, SystolicFFA/1
  SystolicFFB/1 -> OutB/1
  SystolicFFA/1 -> OutA/1
  MulENA/1 -> Mult/1
  MulENB/1 -> Mult/2
  EN/1 -> MulENB/2, MulENA/2
  FFAccum/1 -> AddSub/2
  CLRAccum/1 -> FFAccum/2
  PutPass/1 -> Mux/1
  InS/1 -> Mux/3
  Mux/1 -> OutS/1
  CarryS/1 -> Mux/4

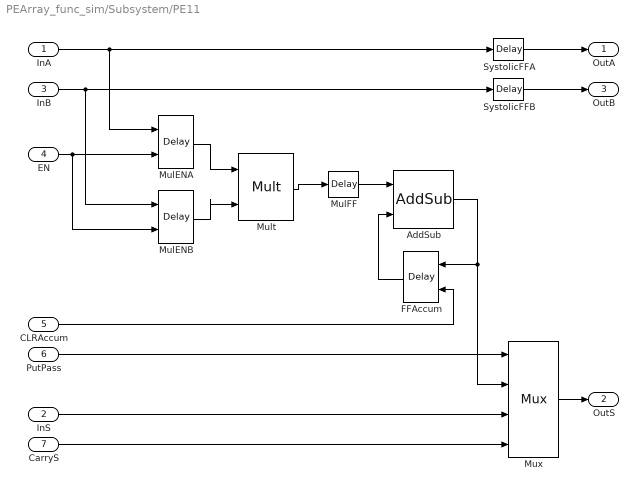
== system PEArray_func_sim/Subsystem/PE11 ==
  InA : Inport
  InS : Inport  Port=2
  InB : Inport  Port=3
  EN : Inport  Port=4
  CLRAccum : Inport  Port=5
  PutPass : Inport  Port=6
  CarryS : Inport  Port=7
  AddSub : hdlBasic/AddSub  mode=Addition  use_carryin=off  use_carryout=off  en=off  latency=0  precision=User Defined  arith_type="Signed  (2's comp)"  n_bits=16  bin_pt=10  quantization=Truncate  overflow=Wrap  use_behavioral_HDL=off  hw_selection=DSP48  pipelined=off  XmcBlockStatus=1  maskContainerNames=tabcontainer1  block_type=addsub  block_config=sysgen:Addsub_config
  FFAccum : hdlBasic/Delay  rst=on  en=off  latency=1  reg_retiming=off  XmcBlockStatus=1  maskContainerNames=group1  block_type=delay  block_config=sysgen:Delay_config
  MulENA : hdlBasic/Delay  rst=on  en=off  latency=1  reg_retiming=off  XmcBlockStatus=1  maskContainerNames=group1  block_type=delay  block_config=sysgen:Delay_config
  MulENB : hdlBasic/Delay  rst=on  en=off  latency=1  reg_retiming=off  XmcBlockStatus=1  maskContainerNames=group1  block_type=delay  block_config=sysgen:Delay_config
  MulFF : hdlBasic/Delay  rst=off  en=off  latency=1  reg_retiming=off  XmcBlockStatus=1  maskContainerNames=group1  block_type=delay  block_config=sysgen:Delay_config
  Mult : hdlBasic/Mult  precision=User Defined  arith_type="Signed  (2's comp)"  n_bits=16  bin_pt=10  quantization=Truncate  overflow=Wrap  en=off  latency=0  use_behavioral_HDL=off  opt=Speed  use_embedded=on  optimum_pipeline=off  pipeline=on  use_rpm=on  placement_style=Triangular  XmcBlockStatus=1  maskContainerNames=group1  block_type=mult  block_config=sysgen:Mult_config
  Mux : hdlBasic/Mux  inputs=2  en=on  latency=1  precision=Full  arith_type=Unsigned  n_bits=16  bin_pt=14  quantization=Truncate  overflow=Wrap  XmcBlockStatus=1  maskContainerNames=tabcontainer1  block_type=mux  block_config=sysgen:Mux_config
  SystolicFFA : hdlBasic/Delay  rst=off  en=off  latency=1  reg_retiming=off  XmcBlockStatus=1  maskContainerNames=group1  block_type=delay  block_config=sysgen:Delay_config
  SystolicFFB : hdlBasic/Delay  rst=off  en=off  latency=1  reg_retiming=off  XmcBlockStatus=1  maskContainerNames=group1  block_type=delay  block_config=sysgen:Delay_config
  OutA : Outport
  OutS : Outport  Port=2
  OutB : Outport  Port=3
  wires:
  Mult/1 -> MulFF/1
  MulFF/1 -> AddSub/1
  AddSub/1 -> Mux/2, FFAccum/1
  InB/1 -> MulENB/1, SystolicFFB/1
  InA/1 -> MulENA/1, SystolicFFA/1
  SystolicFFB/1 -> OutB/1
  SystolicFFA/1 -> OutA/1
  MulENA/1 -> Mult/1
  MulENB/1 -> Mult/2
  EN/1 -> MulENB/2, MulENA/2
  FFAccum/1 -> AddSub/2
  CLRAccum/1 -> FFAccum/2
  PutPass/1 -> Mux/1
  InS/1 -> Mux/3
  Mux/1 -> OutS/1
  CarryS/1 -> Mux/4

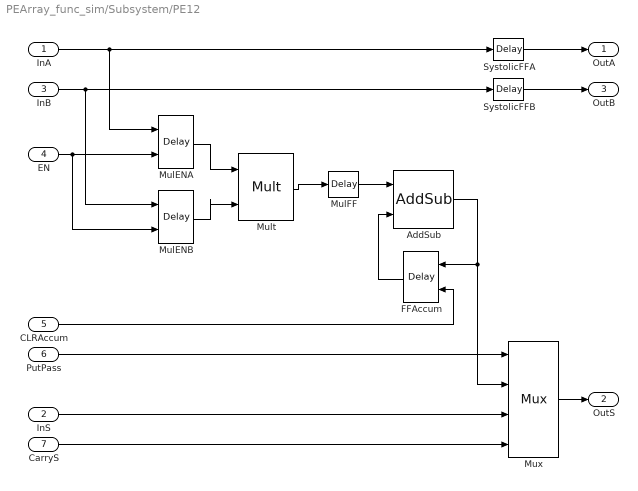
== system PEArray_func_sim/Subsystem/PE12 ==
  InA : Inport
  InS : Inport  Port=2
  InB : Inport  Port=3
  EN : Inport  Port=4
  CLRAccum : Inport  Port=5
  PutPass : Inport  Port=6
  CarryS : Inport  Port=7
  AddSub : hdlBasic/AddSub  mode=Addition  use_carryin=off  use_carryout=off  en=off  latency=0  precision=User Defined  arith_type="Signed  (2's comp)"  n_bits=16  bin_pt=10  quantization=Truncate  overflow=Wrap  use_behavioral_HDL=off  hw_selection=DSP48  pipelined=off  XmcBlockStatus=1  maskContainerNames=tabcontainer1  block_type=addsub  block_config=sysgen:Addsub_config
  FFAccum : hdlBasic/Delay  rst=on  en=off  latency=1  reg_retiming=off  XmcBlockStatus=1  maskContainerNames=group1  block_type=delay  block_config=sysgen:Delay_config
  MulENA : hdlBasic/Delay  rst=on  en=off  latency=1  reg_retiming=off  XmcBlockStatus=1  maskContainerNames=group1  block_type=delay  block_config=sysgen:Delay_config
  MulENB : hdlBasic/Delay  rst=on  en=off  latency=1  reg_retiming=off  XmcBlockStatus=1  maskContainerNames=group1  block_type=delay  block_config=sysgen:Delay_config
  MulFF : hdlBasic/Delay  rst=off  en=off  latency=1  reg_retiming=off  XmcBlockStatus=1  maskContainerNames=group1  block_type=delay  block_config=sysgen:Delay_config
  Mult : hdlBasic/Mult  precision=User Defined  arith_type="Signed  (2's comp)"  n_bits=16  bin_pt=10  quantization=Truncate  overflow=Wrap  en=off  latency=0  use_behavioral_HDL=off  opt=Speed  use_embedded=on  optimum_pipeline=off  pipeline=on  use_rpm=on  placement_style=Triangular  XmcBlockStatus=1  maskContainerNames=group1  block_type=mult  block_config=sysgen:Mult_config
  Mux : hdlBasic/Mux  inputs=2  en=on  latency=1  precision=Full  arith_type=Unsigned  n_bits=16  bin_pt=14  quantization=Truncate  overflow=Wrap  XmcBlockStatus=1  maskContainerNames=tabcontainer1  block_type=mux  block_config=sysgen:Mux_config
  SystolicFFA : hdlBasic/Delay  rst=off  en=off  latency=1  reg_retiming=off  XmcBlockStatus=1  maskContainerNames=group1  block_type=delay  block_config=sysgen:Delay_config
  SystolicFFB : hdlBasic/Delay  rst=off  en=off  latency=1  reg_retiming=off  XmcBlockStatus=1  maskContainerNames=group1  block_type=delay  block_config=sysgen:Delay_config
  OutA : Outport
  OutS : Outport  Port=2
  OutB : Outport  Port=3
  wires:
  Mult/1 -> MulFF/1
  MulFF/1 -> AddSub/1
  AddSub/1 -> Mux/2, FFAccum/1
  InB/1 -> MulENB/1, SystolicFFB/1
  InA/1 -> MulENA/1, SystolicFFA/1
  SystolicFFB/1 -> OutB/1
  SystolicFFA/1 -> OutA/1
  MulENA/1 -> Mult/1
  MulENB/1 -> Mult/2
  EN/1 -> MulENB/2, MulENA/2
  FFAccum/1 -> AddSub/2
  CLRAccum/1 -> FFAccum/2
  PutPass/1 -> Mux/1
  InS/1 -> Mux/3
  Mux/1 -> OutS/1
  CarryS/1 -> Mux/4

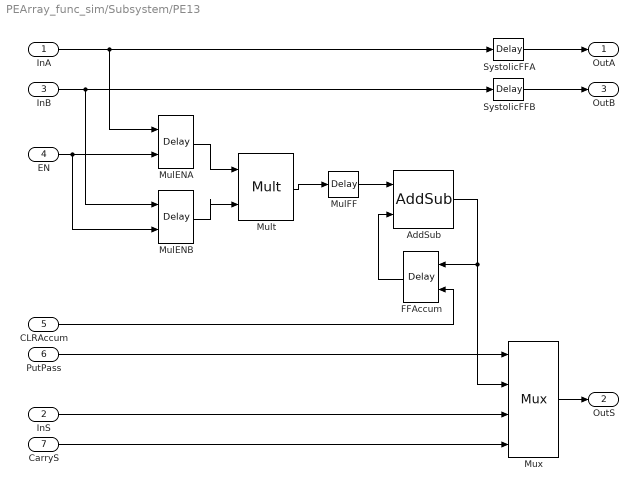
== system PEArray_func_sim/Subsystem/PE13 ==
  InA : Inport
  InS : Inport  Port=2
  InB : Inport  Port=3
  EN : Inport  Port=4
  CLRAccum : Inport  Port=5
  PutPass : Inport  Port=6
  CarryS : Inport  Port=7
  AddSub : hdlBasic/AddSub  mode=Addition  use_carryin=off  use_carryout=off  en=off  latency=0  precision=User Defined  arith_type="Signed  (2's comp)"  n_bits=16  bin_pt=10  quantization=Truncate  overflow=Wrap  use_behavioral_HDL=off  hw_selection=DSP48  pipelined=off  XmcBlockStatus=1  maskContainerNames=tabcontainer1  block_type=addsub  block_config=sysgen:Addsub_config
  FFAccum : hdlBasic/Delay  rst=on  en=off  latency=1  reg_retiming=off  XmcBlockStatus=1  maskContainerNames=group1  block_type=delay  block_config=sysgen:Delay_config
  MulENA : hdlBasic/Delay  rst=on  en=off  latency=1  reg_retiming=off  XmcBlockStatus=1  maskContainerNames=group1  block_type=delay  block_config=sysgen:Delay_config
  MulENB : hdlBasic/Delay  rst=on  en=off  latency=1  reg_retiming=off  XmcBlockStatus=1  maskContainerNames=group1  block_type=delay  block_config=sysgen:Delay_config
  MulFF : hdlBasic/Delay  rst=off  en=off  latency=1  reg_retiming=off  XmcBlockStatus=1  maskContainerNames=group1  block_type=delay  block_config=sysgen:Delay_config
  Mult : hdlBasic/Mult  precision=User Defined  arith_type="Signed  (2's comp)"  n_bits=16  bin_pt=10  quantization=Truncate  overflow=Wrap  en=off  latency=0  use_behavioral_HDL=off  opt=Speed  use_embedded=on  optimum_pipeline=off  pipeline=on  use_rpm=on  placement_style=Triangular  XmcBlockStatus=1  maskContainerNames=group1  block_type=mult  block_config=sysgen:Mult_config
  Mux : hdlBasic/Mux  inputs=2  en=on  latency=1  precision=Full  arith_type=Unsigned  n_bits=16  bin_pt=14  quantization=Truncate  overflow=Wrap  XmcBlockStatus=1  maskContainerNames=tabcontainer1  block_type=mux  block_config=sysgen:Mux_config
  SystolicFFA : hdlBasic/Delay  rst=off  en=off  latency=1  reg_retiming=off  XmcBlockStatus=1  maskContainerNames=group1  block_type=delay  block_config=sysgen:Delay_config
  SystolicFFB : hdlBasic/Delay  rst=off  en=off  latency=1  reg_retiming=off  XmcBlockStatus=1  maskContainerNames=group1  block_type=delay  block_config=sysgen:Delay_config
  OutA : Outport
  OutS : Outport  Port=2
  OutB : Outport  Port=3
  wires:
  Mult/1 -> MulFF/1
  MulFF/1 -> AddSub/1
  AddSub/1 -> Mux/2, FFAccum/1
  InB/1 -> MulENB/1, SystolicFFB/1
  InA/1 -> MulENA/1, SystolicFFA/1
  SystolicFFB/1 -> OutB/1
  SystolicFFA/1 -> OutA/1
  MulENA/1 -> Mult/1
  MulENB/1 -> Mult/2
  EN/1 -> MulENB/2, MulENA/2
  FFAccum/1 -> AddSub/2
  CLRAccum/1 -> FFAccum/2
  PutPass/1 -> Mux/1
  InS/1 -> Mux/3
  Mux/1 -> OutS/1
  CarryS/1 -> Mux/4

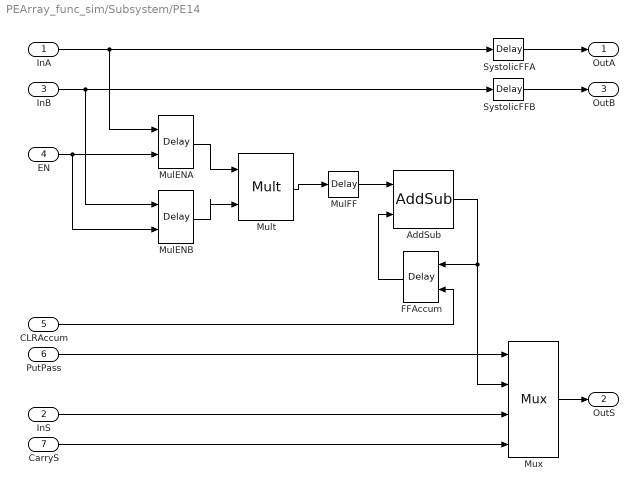
== system PEArray_func_sim/Subsystem/PE14 ==
  InA : Inport
  InS : Inport  Port=2
  InB : Inport  Port=3
  EN : Inport  Port=4
  CLRAccum : Inport  Port=5
  PutPass : Inport  Port=6
  CarryS : Inport  Port=7
  AddSub : hdlBasic/AddSub  mode=Addition  use_carryin=off  use_carryout=off  en=off  latency=0  precision=User Defined  arith_type="Signed  (2's comp)"  n_bits=16  bin_pt=10  quantization=Truncate  overflow=Wrap  use_behavioral_HDL=off  hw_selection=DSP48  pipelined=off  XmcBlockStatus=1  maskContainerNames=tabcontainer1  block_type=addsub  block_config=sysgen:Addsub_config
  FFAccum : hdlBasic/Delay  rst=on  en=off  latency=1  reg_retiming=off  XmcBlockStatus=1  maskContainerNames=group1  block_type=delay  block_config=sysgen:Delay_config
  MulENA : hdlBasic/Delay  rst=on  en=off  latency=1  reg_retiming=off  XmcBlockStatus=1  maskContainerNames=group1  block_type=delay  block_config=sysgen:Delay_config
  MulENB : hdlBasic/Delay  rst=on  en=off  latency=1  reg_retiming=off  XmcBlockStatus=1  maskContainerNames=group1  block_type=delay  block_config=sysgen:Delay_config
  MulFF : hdlBasic/Delay  rst=off  en=off  latency=1  reg_retiming=off  XmcBlockStatus=1  maskContainerNames=group1  block_type=delay  block_config=sysgen:Delay_config
  Mult : hdlBasic/Mult  precision=User Defined  arith_type="Signed  (2's comp)"  n_bits=16  bin_pt=10  quantization=Truncate  overflow=Wrap  en=off  latency=0  use_behavioral_HDL=off  opt=Speed  use_embedded=on  optimum_pipeline=off  pipeline=on  use_rpm=on  placement_style=Triangular  XmcBlockStatus=1  maskContainerNames=group1  block_type=mult  block_config=sysgen:Mult_config
  Mux : hdlBasic/Mux  inputs=2  en=on  latency=1  precision=Full  arith_type=Unsigned  n_bits=16  bin_pt=14  quantization=Truncate  overflow=Wrap  XmcBlockStatus=1  maskContainerNames=tabcontainer1  block_type=mux  block_config=sysgen:Mux_config
  SystolicFFA : hdlBasic/Delay  rst=off  en=off  latency=1  reg_retiming=off  XmcBlockStatus=1  maskContainerNames=group1  block_type=delay  block_config=sysgen:Delay_config
  SystolicFFB : hdlBasic/Delay  rst=off  en=off  latency=1  reg_retiming=off  XmcBlockStatus=1  maskContainerNames=group1  block_type=delay  block_config=sysgen:Delay_config
  OutA : Outport
  OutS : Outport  Port=2
  OutB : Outport  Port=3
  wires:
  Mult/1 -> MulFF/1
  MulFF/1 -> AddSub/1
  AddSub/1 -> Mux/2, FFAccum/1
  InB/1 -> MulENB/1, SystolicFFB/1
  InA/1 -> MulENA/1, SystolicFFA/1
  SystolicFFB/1 -> OutB/1
  SystolicFFA/1 -> OutA/1
  MulENA/1 -> Mult/1
  MulENB/1 -> Mult/2
  EN/1 -> MulENB/2, MulENA/2
  FFAccum/1 -> AddSub/2
  CLRAccum/1 -> FFAccum/2
  PutPass/1 -> Mux/1
  InS/1 -> Mux/3
  Mux/1 -> OutS/1
  CarryS/1 -> Mux/4

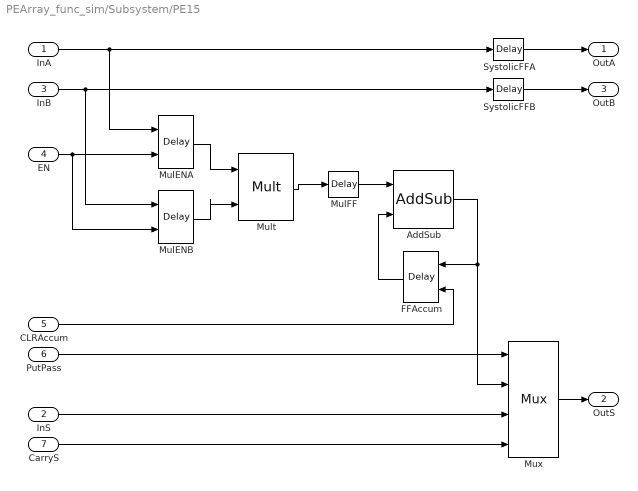
== system PEArray_func_sim/Subsystem/PE15 ==
  InA : Inport
  InS : Inport  Port=2
  InB : Inport  Port=3
  EN : Inport  Port=4
  CLRAccum : Inport  Port=5
  PutPass : Inport  Port=6
  CarryS : Inport  Port=7
  AddSub : hdlBasic/AddSub  mode=Addition  use_carryin=off  use_carryout=off  en=off  latency=0  precision=User Defined  arith_type="Signed  (2's comp)"  n_bits=16  bin_pt=10  quantization=Truncate  overflow=Wrap  use_behavioral_HDL=off  hw_selection=DSP48  pipelined=off  XmcBlockStatus=1  maskContainerNames=tabcontainer1  block_type=addsub  block_config=sysgen:Addsub_config
  FFAccum : hdlBasic/Delay  rst=on  en=off  latency=1  reg_retiming=off  XmcBlockStatus=1  maskContainerNames=group1  block_type=delay  block_config=sysgen:Delay_config
  MulENA : hdlBasic/Delay  rst=on  en=off  latency=1  reg_retiming=off  XmcBlockStatus=1  maskContainerNames=group1  block_type=delay  block_config=sysgen:Delay_config
  MulENB : hdlBasic/Delay  rst=on  en=off  latency=1  reg_retiming=off  XmcBlockStatus=1  maskContainerNames=group1  block_type=delay  block_config=sysgen:Delay_config
  MulFF : hdlBasic/Delay  rst=off  en=off  latency=1  reg_retiming=off  XmcBlockStatus=1  maskContainerNames=group1  block_type=delay  block_config=sysgen:Delay_config
  Mult : hdlBasic/Mult  precision=User Defined  arith_type="Signed  (2's comp)"  n_bits=16  bin_pt=10  quantization=Truncate  overflow=Wrap  en=off  latency=0  use_behavioral_HDL=off  opt=Speed  use_embedded=on  optimum_pipeline=off  pipeline=on  use_rpm=on  placement_style=Triangular  XmcBlockStatus=1  maskContainerNames=group1  block_type=mult  block_config=sysgen:Mult_config
  Mux : hdlBasic/Mux  inputs=2  en=on  latency=1  precision=Full  arith_type=Unsigned  n_bits=16  bin_pt=14  quantization=Truncate  overflow=Wrap  XmcBlockStatus=1  maskContainerNames=tabcontainer1  block_type=mux  block_config=sysgen:Mux_config
  SystolicFFA : hdlBasic/Delay  rst=off  en=off  latency=1  reg_retiming=off  XmcBlockStatus=1  maskContainerNames=group1  block_type=delay  block_config=sysgen:Delay_config
  SystolicFFB : hdlBasic/Delay  rst=off  en=off  latency=1  reg_retiming=off  XmcBlockStatus=1  maskContainerNames=group1  block_type=delay  block_config=sysgen:Delay_config
  OutA : Outport
  OutS : Outport  Port=2
  OutB : Outport  Port=3
  wires:
  Mult/1 -> MulFF/1
  MulFF/1 -> AddSub/1
  AddSub/1 -> Mux/2, FFAccum/1
  InB/1 -> MulENB/1, SystolicFFB/1
  InA/1 -> MulENA/1, SystolicFFA/1
  SystolicFFB/1 -> OutB/1
  SystolicFFA/1 -> OutA/1
  MulENA/1 -> Mult/1
  MulENB/1 -> Mult/2
  EN/1 -> MulENB/2, MulENA/2
  FFAccum/1 -> AddSub/2
  CLRAccum/1 -> FFAccum/2
  PutPass/1 -> Mux/1
  InS/1 -> Mux/3
  Mux/1 -> OutS/1
  CarryS/1 -> Mux/4

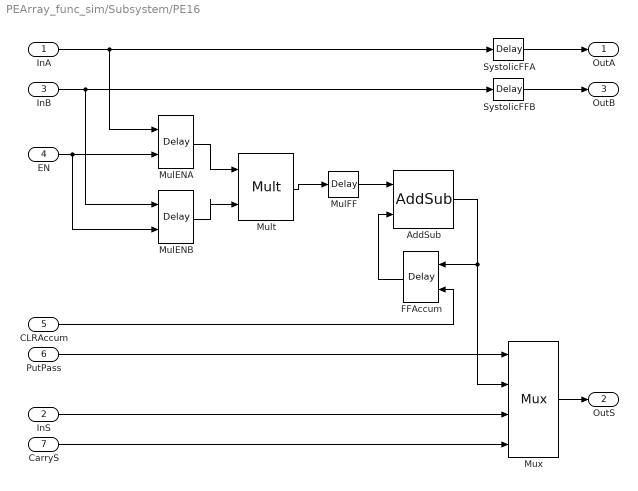
== system PEArray_func_sim/Subsystem/PE16 ==
  InA : Inport
  InS : Inport  Port=2
  InB : Inport  Port=3
  EN : Inport  Port=4
  CLRAccum : Inport  Port=5
  PutPass : Inport  Port=6
  CarryS : Inport  Port=7
  AddSub : hdlBasic/AddSub  mode=Addition  use_carryin=off  use_carryout=off  en=off  latency=0  precision=User Defined  arith_type="Signed  (2's comp)"  n_bits=16  bin_pt=10  quantization=Truncate  overflow=Wrap  use_behavioral_HDL=off  hw_selection=DSP48  pipelined=off  XmcBlockStatus=1  maskContainerNames=tabcontainer1  block_type=addsub  block_config=sysgen:Addsub_config
  FFAccum : hdlBasic/Delay  rst=on  en=off  latency=1  reg_retiming=off  XmcBlockStatus=1  maskContainerNames=group1  block_type=delay  block_config=sysgen:Delay_config
  MulENA : hdlBasic/Delay  rst=on  en=off  latency=1  reg_retiming=off  XmcBlockStatus=1  maskContainerNames=group1  block_type=delay  block_config=sysgen:Delay_config
  MulENB : hdlBasic/Delay  rst=on  en=off  latency=1  reg_retiming=off  XmcBlockStatus=1  maskContainerNames=group1  block_type=delay  block_config=sysgen:Delay_config
  MulFF : hdlBasic/Delay  rst=off  en=off  latency=1  reg_retiming=off  XmcBlockStatus=1  maskContainerNames=group1  block_type=delay  block_config=sysgen:Delay_config
  Mult : hdlBasic/Mult  precision=User Defined  arith_type="Signed  (2's comp)"  n_bits=16  bin_pt=10  quantization=Truncate  overflow=Wrap  en=off  latency=0  use_behavioral_HDL=off  opt=Speed  use_embedded=on  optimum_pipeline=off  pipeline=on  use_rpm=on  placement_style=Triangular  XmcBlockStatus=1  maskContainerNames=group1  block_type=mult  block_config=sysgen:Mult_config
  Mux : hdlBasic/Mux  inputs=2  en=on  latency=1  precision=Full  arith_type=Unsigned  n_bits=16  bin_pt=14  quantization=Truncate  overflow=Wrap  XmcBlockStatus=1  maskContainerNames=tabcontainer1  block_type=mux  block_config=sysgen:Mux_config
  SystolicFFA : hdlBasic/Delay  rst=off  en=off  latency=1  reg_retiming=off  XmcBlockStatus=1  maskContainerNames=group1  block_type=delay  block_config=sysgen:Delay_config
  SystolicFFB : hdlBasic/Delay  rst=off  en=off  latency=1  reg_retiming=off  XmcBlockStatus=1  maskContainerNames=group1  block_type=delay  block_config=sysgen:Delay_config
  OutA : Outport
  OutS : Outport  Port=2
  OutB : Outport  Port=3
  wires:
  Mult/1 -> MulFF/1
  MulFF/1 -> AddSub/1
  AddSub/1 -> Mux/2, FFAccum/1
  InB/1 -> MulENB/1, SystolicFFB/1
  InA/1 -> MulENA/1, SystolicFFA/1
  SystolicFFB/1 -> OutB/1
  SystolicFFA/1 -> OutA/1
  MulENA/1 -> Mult/1
  MulENB/1 -> Mult/2
  EN/1 -> MulENB/2, MulENA/2
  FFAccum/1 -> AddSub/2
  CLRAccum/1 -> FFAccum/2
  PutPass/1 -> Mux/1
  InS/1 -> Mux/3
  Mux/1 -> OutS/1
  CarryS/1 -> Mux/4
